simulink model "sampleModel1771"  (R2023a)
settings: Solver=VariableStepAuto  StartTime=0.0  StopTime=10.0  RelTol=1e-3
libraries: hdlsllib x4
settings Model: Creator=user1  LastModifiedBy=user1

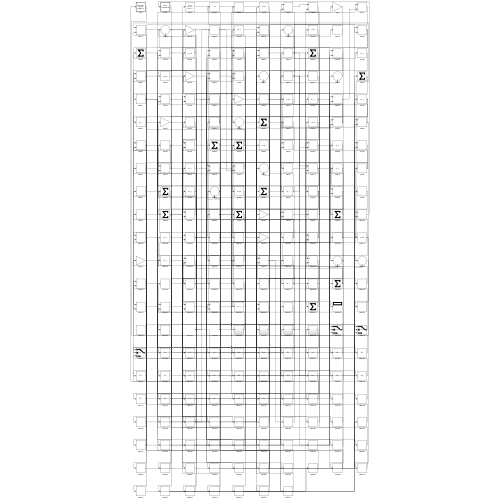
[thumbnail: Simulink's stored preview of the top-level diagram]
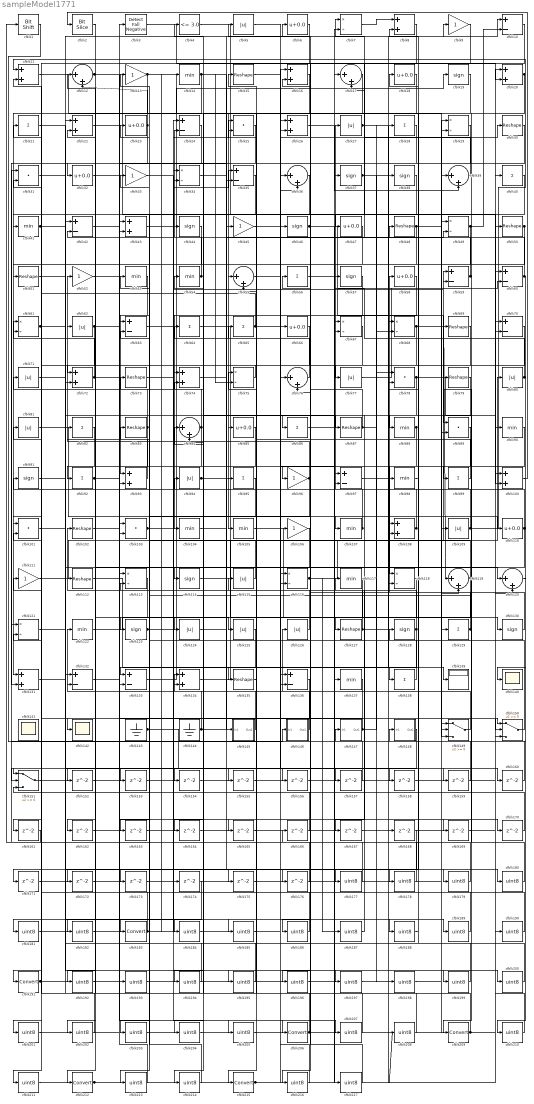
== system sampleModel1771 ==
  cfblk1 : hdlsllib/Logic and Bit Operations/Bit Shift  mode=Shift Left Logical  N=0
  cfblk{10,24,35,42,59..60,63,70,97,132..133,136} (12 alike) : Sum  Inputs=+-
  cfblk{8,11,16,20,22,26,43,72,74,93,100,108,131,134} (14 alike) : Sum
  cfblk{25,31,78,89,101,103} (6 alike) : DotProduct  OutDataTypeStr=Inherit: Inherit via internal rule
  cfblk{15,30,48,50..51,69,73,79,83,87,102,112,127,135} (14 alike) : Reshape
  cfblk{14,41,53..54,88,90,98,104..105,107,117,122,137} (13 alike) : MinMax
  cfblk{9,13,33,45,52,96,106,111} (8 alike) : Gain
  cfblk{5,27,62,71,77,80..81,94,109,115,124..126} (13 alike) : Abs  SaturateOnIntegerOverflow=off
  cfblk{6,18,23,32,47,58,66,85,110} (9 alike) : Bias  Bias=0.0  SaturateOnIntegerOverflow=off
  cfblk{7,29,34,49,61,67..68,75,113,116,118,121} (12 alike) : Product  Inputs=*/  RndMeth=Zero  SaturateOnIntegerOverflow=on
  cfblk{19,37..38,44,46,57,91,114,123,128,130} (11 alike) : Signum
  cfblk{12,17,36,39,55,76,84,119..120} (9 alike) : Sum  Inputs=|++
  cfblk{21,28,40,56,64..65,82,86,92,95,99,129,138} (13 alike) : Sum  Inputs=+
  cfblk139 : Display
  cfblk140 : Scope
  cfblk141 : Scope
      settings: Floating=on
  cfblk142 : Scope
  cfblk143 : Ground
  cfblk144 : Ground
  cfblk145 : Subsystem
      settings: LibrarySourceBlock=|
      | hdlsllib/Ports &
      | Subsystems/Subsystem
  cfblk146 : Subsystem
      settings: LibrarySourceBlock=|
      | hdlsllib/Ports &
      | Subsystems/Subsystem
  cfblk147 : Subsystem
      settings: LibrarySourceBlock=|
      | hdlsllib/Ports &
      | Subsystems/Subsystem
  cfblk148 : Subsystem
      settings: LibrarySourceBlock=|
      | hdlsllib/Ports &
      | Subsystems/Subsystem
  cfblk149 : Switch  SaturateOnIntegerOverflow=off  InputSameDT=off
  cfblk150 : Switch  SaturateOnIntegerOverflow=off  InputSameDT=off
  cfblk151 : Switch  SaturateOnIntegerOverflow=off  InputSameDT=off
  cfblk{152..176} (25 alike) : Delay  SampleTime=1
  cfblk{177..182,184..190,192..205,207..208,210..211,213..214,216..217} (35 alike) : DataTypeConversion  OutDataTypeStr=uint8  SaturateOnIntegerOverflow=off  RndMeth=Floor
  cfblk{183,191,206,209,212,215} (6 alike) : DataTypeConversion  SaturateOnIntegerOverflow=off  RndMeth=Floor
  cfblk2 : hdlsllib/Logic and Bit Operations/Bit Slice  lidx=7  ridx=0
  cfblk3 : hdlsllib/Logic and Bit Operations/Detect Fall Negative  vinit=0  OutDataTypeStr=boolean
  cfblk4 : hdlsllib/Logic and Bit Operations/Compare To Constant  relop=<=  const=3.0  OutDataTypeStr=boolean
  wires:
  cfblk36/1 -> cfblk183/1
  cfblk13/1 -> cfblk131/1, cfblk106/1
  cfblk133/1 -> cfblk19/1
  cfblk23/1 -> cfblk32/1, cfblk12/2
  cfblk107/1 -> cfblk27/1, cfblk81/1
  cfblk146/1(Out1) -> cfblk126/1
  cfblk92/1 -> cfblk165/1, cfblk179/1
  cfblk109/1 -> cfblk11/1, cfblk74/2, cfblk78/2
  cfblk64/1 -> cfblk130/1
  cfblk24/1 -> cfblk131/2
  cfblk58/1 -> cfblk104/1
  cfblk53/1 -> cfblk93/1
  cfblk60/1 -> cfblk17/2, cfblk210/1
  cfblk108/1 -> cfblk53/1, cfblk94/1
  cfblk145/1(Out1) -> cfblk122/1
  cfblk31/1 -> cfblk87/1
  cfblk86/1 -> cfblk17/1
  cfblk3/1 -> cfblk20/2
  cfblk76/1 -> cfblk64/1
  cfblk12/1 -> cfblk105/1, cfblk35/2
  cfblk113/1 -> cfblk212/1
  cfblk126/1 -> cfblk102/1
  cfblk20/1 -> cfblk55/1, cfblk99/1
  cfblk115/1 -> cfblk83/1
  cfblk137/1 -> cfblk191/1
  cfblk1/1 -> cfblk146/1(In1)
  cfblk149/1 -> cfblk134/1
  cfblk111/1 -> cfblk45/1
  cfblk63/1 -> cfblk59/1
  cfblk83/1 -> cfblk61/1, cfblk172/1
  cfblk99/1 -> cfblk55/2
  cfblk129/1 -> cfblk58/1, cfblk73/1
  cfblk68/1 -> cfblk119/1, cfblk77/1
  cfblk151/1 -> cfblk136/1
  cfblk81/1 -> cfblk149/1
  cfblk39/1 -> cfblk7/1
  cfblk134/1 -> cfblk59/2
  cfblk147/1(Out1) -> cfblk142/1, cfblk68/2
  cfblk10/1 -> cfblk96/1
  cfblk67/1 -> cfblk124/1
  cfblk69/1 -> cfblk93/2
  cfblk54/1 -> cfblk51/1, cfblk12/1
  cfblk100/1 -> cfblk2/1
  cfblk114/1 -> cfblk80/1
  cfblk102/1 -> cfblk3/1
  cfblk4/1 -> cfblk100/1
  cfblk105/1 -> cfblk149/2
  cfblk106/1 -> cfblk133/1
  cfblk94/1 -> cfblk107/1, cfblk169/1
  cfblk135/1 -> cfblk65/1
  cfblk122/1 -> cfblk125/1
  cfblk49/1 -> cfblk88/1, cfblk10/2
  cfblk50/1 -> cfblk85/1, cfblk175/1
  cfblk46/1 -> cfblk89/1, cfblk170/1
  cfblk87/1 -> cfblk5/1, cfblk38/1
  cfblk112/1 -> cfblk138/1
  cfblk82/1 -> cfblk92/1
  cfblk70/1 -> cfblk209/1
  cfblk14/1 -> cfblk133/2, cfblk136/2, cfblk75/2
  cfblk97/1 -> cfblk118/1
  cfblk77/1 -> cfblk49/1
  cfblk89/1 -> cfblk98/1
  cfblk123/1 -> cfblk108/2, cfblk197/1
  cfblk93/1 -> cfblk52/1
  cfblk144/1 -> cfblk112/1, cfblk10/1
  cfblk62/1 -> cfblk101/1, cfblk184/1
  cfblk88/1 -> cfblk135/1, cfblk163/1
  cfblk91/1 -> cfblk6/1
  cfblk79/1 -> cfblk114/1
  cfblk37/1 -> cfblk78/1, cfblk198/1
  cfblk120/1 -> cfblk147/1(In1)
  cfblk16/1 -> cfblk215/1
  cfblk128/1 -> cfblk134/2, cfblk63/2
  cfblk32/1 -> cfblk149/3
  cfblk138/1 -> cfblk128/1
  cfblk124/1 -> cfblk49/2
  cfblk98/1 -> cfblk18/1
  cfblk27/1 -> cfblk139/1, cfblk168/1
  cfblk65/1 -> cfblk21/1, cfblk127/1
  cfblk150/1 -> cfblk33/1
  cfblk59/1 -> cfblk24/2, cfblk15/1
  cfblk41/1 -> cfblk86/1, cfblk173/1
  cfblk84/1 -> cfblk62/1, cfblk103/2
  cfblk44/1 -> cfblk63/1
  cfblk103/1 -> cfblk150/1, cfblk35/1, cfblk25/1
  cfblk75/1 -> cfblk74/1
  cfblk26/1 -> cfblk39/2
  cfblk7/1 -> cfblk8/1
  cfblk78/1 -> cfblk100/2, cfblk167/1
  cfblk127/1 -> cfblk23/1, cfblk9/1
  cfblk101/1 -> cfblk120/1
  cfblk42/1 -> cfblk206/1
  cfblk56/1 -> cfblk60/2
  cfblk5/1 -> cfblk97/2
  cfblk130/1 -> cfblk56/1
  cfblk96/1 -> cfblk82/1, cfblk164/1
  cfblk11/1 -> cfblk89/2
  cfblk61/1 -> cfblk151/1, cfblk185/1
  cfblk110/1 -> cfblk140/1, cfblk75/1, cfblk182/1
  cfblk45/1 -> cfblk30/1
  cfblk148/1(Out1) -> cfblk151/2
  cfblk119/1 -> cfblk54/1, cfblk192/1
  cfblk66/1 -> cfblk123/1
  cfblk30/1 -> cfblk41/1
  cfblk80/1 -> cfblk57/1, cfblk72/1
  cfblk116/1 -> cfblk69/1, cfblk187/1
  cfblk72/1 -> cfblk31/2, cfblk150/2
  cfblk48/1 -> cfblk110/1, cfblk72/2
  cfblk8/1 -> cfblk76/2
  cfblk55/1 -> cfblk26/2
  cfblk104/1 -> cfblk108/1
  cfblk74/1 -> cfblk145/1(In1)
  cfblk9/1 -> cfblk47/1
  cfblk17/1 -> cfblk95/1
  cfblk143/1 -> cfblk13/1, cfblk14/1, cfblk217/1
  cfblk2/1 -> cfblk152/1
  cfblk152/1 -> cfblk60/1
  cfblk125/1 -> cfblk153/1
  cfblk57/1 -> cfblk154/1
  cfblk154/1 -> cfblk26/1
  cfblk28/1 -> cfblk155/1
  cfblk155/1 -> cfblk97/1
  cfblk52/1 -> cfblk156/1
  cfblk71/1 -> cfblk157/1
  cfblk157/1 -> cfblk31/1
  cfblk21/1 -> cfblk158/1
  cfblk158/1 -> cfblk8/2
  cfblk131/1 -> cfblk159/1
  cfblk159/1 -> cfblk24/1
  cfblk15/1 -> cfblk160/1
  cfblk160/1 -> cfblk67/1
  cfblk35/1 -> cfblk161/1
  cfblk161/1 -> cfblk1/1
  cfblk47/1 -> cfblk162/1
  cfblk162/1 -> cfblk119/2
  cfblk163/1 -> cfblk7/2
  cfblk164/1 -> cfblk84/1
  cfblk165/1 -> cfblk20/1
  cfblk166/1 -> cfblk151/3
  cfblk167/1 -> cfblk68/1
  cfblk169/1 -> cfblk120/2
  cfblk170/1 -> cfblk61/2
  cfblk25/1 -> cfblk171/1
  cfblk171/1 -> cfblk76/1
  cfblk172/1 -> cfblk118/2
  cfblk73/1 -> cfblk174/1
  cfblk175/1 -> cfblk39/1
  cfblk38/1 -> cfblk176/1
  cfblk176/1 -> cfblk101/2
  cfblk121/1 -> cfblk177/1
  cfblk177/1 -> cfblk166/1
  cfblk19/1 -> cfblk178/1
  cfblk178/1 -> cfblk121/1
  cfblk179/1 -> cfblk121/2
  cfblk34/1 -> cfblk180/1
  cfblk180/1 -> cfblk79/1
  cfblk168/1 -> cfblk181/1
  cfblk181/1 -> cfblk34/1
  cfblk182/1 -> cfblk34/2
  cfblk183/1 -> cfblk103/1, cfblk44/1, cfblk66/1
  cfblk184/1 -> cfblk36/1
  cfblk185/1 -> cfblk36/2
  cfblk117/1 -> cfblk186/1
  cfblk186/1 -> cfblk71/1
  cfblk187/1 -> cfblk117/1
  cfblk22/1 -> cfblk188/1
  cfblk188/1 -> cfblk148/1(In1)
  cfblk156/1 -> cfblk189/1
  cfblk189/1 -> cfblk22/1
  cfblk190/1 -> cfblk22/2
  cfblk191/1 -> cfblk116/2, cfblk91/1
  cfblk192/1 -> cfblk137/1
  cfblk132/1 -> cfblk193/1
  cfblk193/1 -> cfblk37/1
  cfblk136/1 -> cfblk194/1
  cfblk194/1 -> cfblk132/1
  cfblk51/1 -> cfblk195/1
  cfblk195/1 -> cfblk132/2
  cfblk29/1 -> cfblk196/1
  cfblk196/1 -> cfblk109/1
  cfblk197/1 -> cfblk29/1
  cfblk198/1 -> cfblk29/2
  cfblk43/1 -> cfblk199/1
  cfblk199/1 -> cfblk48/1
  cfblk153/1 -> cfblk200/1
  cfblk200/1 -> cfblk43/1
  cfblk6/1 -> cfblk201/1
  cfblk201/1 -> cfblk43/2
  cfblk90/1 -> cfblk202/1
  cfblk202/1 -> cfblk11/2
  cfblk85/1 -> cfblk203/1
  cfblk203/1 -> cfblk90/1
  cfblk40/1 -> cfblk204/1
  cfblk204/1 -> cfblk46/1
  cfblk33/1 -> cfblk205/1
  cfblk205/1 -> cfblk40/1
  cfblk206/1 -> cfblk25/2, cfblk129/1, cfblk111/1, cfblk115/1
  cfblk173/1 -> cfblk207/1
  cfblk207/1 -> cfblk42/1
  cfblk208/1 -> cfblk42/2
  cfblk209/1 -> cfblk150/3, cfblk84/2, cfblk4/1
  cfblk210/1 -> cfblk70/1
  cfblk174/1 -> cfblk211/1
  cfblk211/1 -> cfblk70/2
  cfblk212/1 -> cfblk67/2, cfblk116/1, cfblk28/1
  cfblk95/1 -> cfblk213/1
  cfblk213/1 -> cfblk113/1
  cfblk18/1 -> cfblk214/1
  cfblk214/1 -> cfblk113/2
  cfblk215/1 -> cfblk208/1, cfblk190/1, cfblk50/1
  cfblk118/1 -> cfblk216/1
  cfblk216/1 -> cfblk16/1
  cfblk217/1 -> cfblk16/2

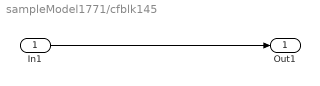
== system sampleModel1771/cfblk145 ==
  In1 : Inport
  Out1 : Outport
  wires:
  In1/1 -> Out1/1

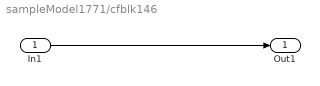
== system sampleModel1771/cfblk146 ==
  In1 : Inport
  Out1 : Outport
  wires:
  In1/1 -> Out1/1

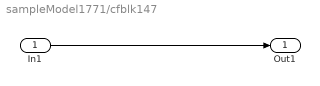
== system sampleModel1771/cfblk147 ==
  In1 : Inport
  Out1 : Outport
  wires:
  In1/1 -> Out1/1

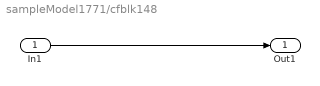
== system sampleModel1771/cfblk148 ==
  In1 : Inport
  Out1 : Outport
  wires:
  In1/1 -> Out1/1
